simulink model "sinwareGain"  (R2017a)
settings: Solver=VariableStepAuto  StartTime=0.0  StopTime=10.0  RelTol=1e-3
settings Model: Creator=Administrator  LastModifiedBy=Administrator

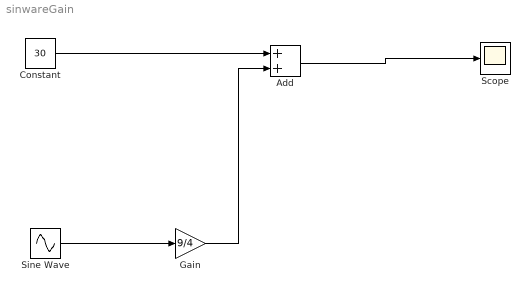
== system sinwareGain ==
  Add : Sum
  Constant : Constant  Value=30
  Gain : Gain  Gain=9/4
  Scope : Scope
  Sine Wave : Sin  SampleTime=0
  wires:
  Constant/1 -> Add/1
  Add/1 -> Scope/1
  Sine Wave/1 -> Gain/1
  Gain/1 -> Add/2
